simulink model "nonlinearGFLcontrol_shell"  (R2023b)
settings: Solver=VariableStepAuto  StartTime=0.0  StopTime=10.0  RelTol=1e-3
undefined symbols (not defined in the file or in its folder): freq, Ki_CC, ki_PLL, Kp_CC, kp_PLL, Lconv1
settings Model: Creator=weq968  LastModifiedBy=kauchr
settings DataIOCC: LoadExternalInput=on
settings RTWCC: GPUComputeCapability=5.0

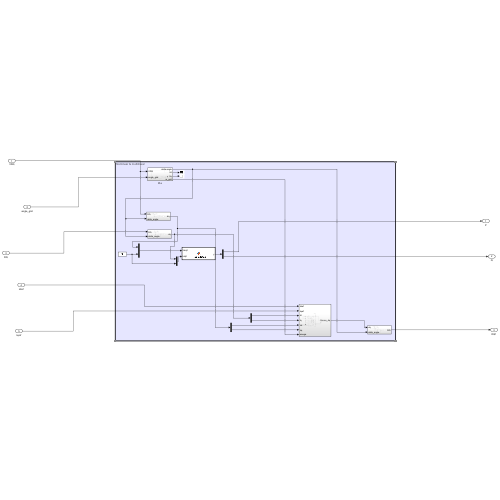
[thumbnail: Simulink's stored preview of the top-level diagram]
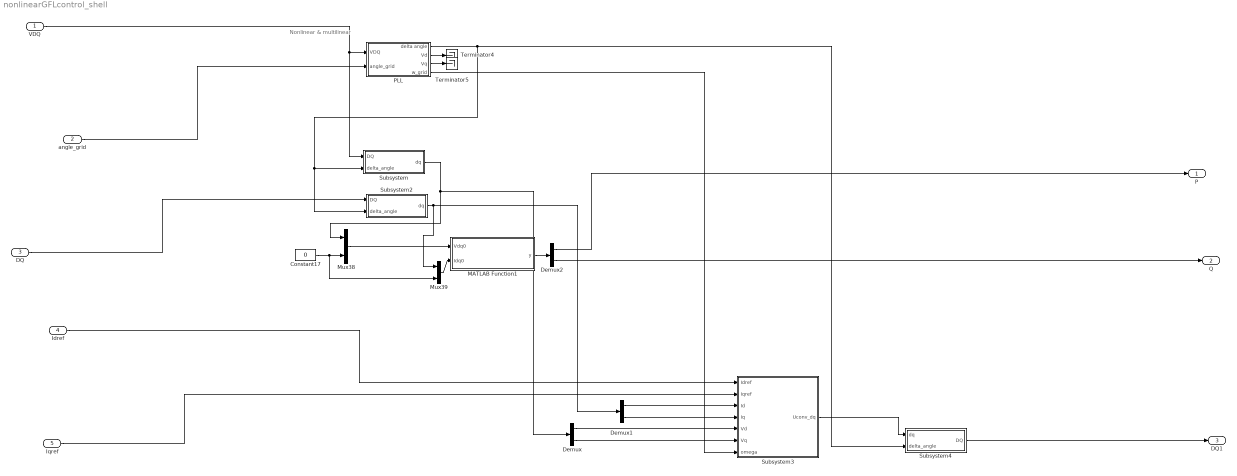
== system nonlinearGFLcontrol_shell ==
  note: Nonlinear & multilinear
  VDQ : Inport
  angle_grid : Inport  Port=2
  DQ : Inport  Port=3
  Idref : Inport  Port=4
  Iqref : Inport  Port=5
  Constant17 : Constant  Value=0
  Demux : Demux  Outputs=2
  Demux1 : Demux  Outputs=2
  Demux2 : Demux  Outputs=2
  MATLAB Function1 : MATLAB Function  TreatAsAtomicUnit=on
  Mux38 : Mux  Inputs=[2 1]
  Mux39 : Mux  Inputs=[2 1]
  PLL : Subsystem
  Subsystem : Subsystem
  Subsystem2 : Subsystem
  Subsystem3 : Subsystem
  Subsystem4 : Subsystem
  Terminator4 : Terminator
  Terminator5 : Terminator
  P : Outport
  Q : Outport  Port=2
  DQ1 : Outport  Port=3
  wires:
  Demux/1 -> Subsystem3/5(Vd)
  Demux1/1 -> Subsystem3/3(Id)
  PLL/4(w_grid) -> Subsystem3/7(omega)
  Subsystem3/1(Uconv_dq) -> Subsystem4/1(dq)
  PLL/2(Vd) -> Terminator4/1
  Iqref/1 -> Subsystem3/2(Iqref)
  Demux2/2 -> Q/1
  Subsystem4/1(DQ) -> DQ1/1
  Idref/1 -> Subsystem3/1(Idref)
  DQ/1 -> Subsystem2/1(DQ)
  Demux1/2 -> Subsystem3/4(Iq)
  Subsystem/1(dq) -> Mux38/1, Demux/1
  Subsystem2/1(dq) -> Mux39/1, Demux1/1
  angle_grid/1 -> PLL/2(angle_grid)
  PLL/1(delta angle) -> Subsystem2/2(delta_angle), Subsystem/2(delta_angle), Subsystem4/2(delta_angle)
  Constant17/1 -> Mux39/2, Mux38/2
  Demux/2 -> Subsystem3/6(Vq)
  VDQ/1 -> Subsystem/1(DQ), PLL/1(VDQ)
  Demux2/1 -> P/1
  Mux39/1 -> MATLAB Function1/2(Idq0)
  Mux38/1 -> MATLAB Function1/1(Vdq0)
  PLL/3(Vq) -> Terminator5/1
  MATLAB Function1/1(y) -> Demux2/1

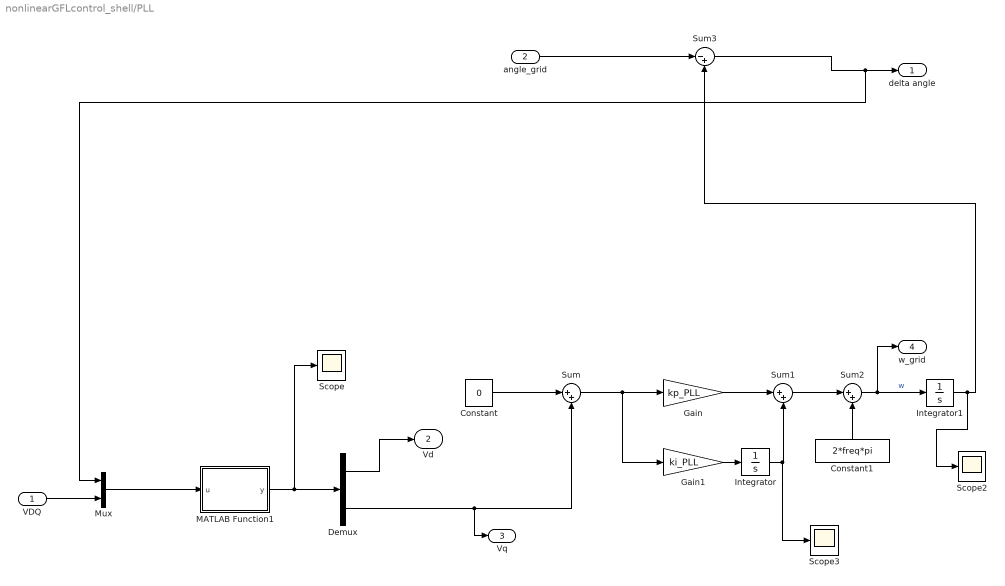
== system nonlinearGFLcontrol_shell/PLL ==
  VDQ : Inport
  angle_grid : Inport  Port=2
  Constant : Constant  Value=0
  Constant1 : Constant  Value=2*freq*pi
  Demux : Demux  Outputs=2
  Gain : Gain  Gain=kp_PLL
  Gain1 : Gain  Gain=ki_PLL
  Integrator : Integrator  ContinuousStateAttributes='converter2_xI_PLL'
  Integrator1 : Integrator  ContinuousStateAttributes='converter2_thetaPLL'
  MATLAB Function1 : MATLAB Function  TreatAsAtomicUnit=on
  Mux : Mux  Inputs=[1 2]
  Scope : Scope
  Scope2 : Scope
  Scope3 : Scope
  Sum : Sum  Inputs=|++
  Sum1 : Sum  Inputs=|++
  Sum2 : Sum  Inputs=|++
  Sum3 : Sum  Inputs=|-+
  delta angle : Outport
  Vd : Outport  Port=2
  Vq : Outport  Port=3
  w_grid : Outport  Port=4
  wires:
  Sum1/1 -> Sum2/1
  Gain/1 -> Sum1/1
  Integrator/1 -> Scope3/1, Sum1/2
  Gain1/1 -> Integrator/1
  Demux/1 -> Vd/1
  Sum2/1 -> w_grid/1, Integrator1/1  "w"
  Constant/1 -> Sum/1
  Constant1/1 -> Sum2/2
  MATLAB Function1/1(y) -> Scope/1, Demux/1
  VDQ/1 -> Mux/2
  Sum/1 -> Gain1/1, Gain/1
  Mux/1 -> MATLAB Function1/1(u)
  Demux/2 -> Vq/1, Sum/2
  Integrator1/1 -> Scope2/1, Sum3/2
  Sum3/1 -> Mux/1, delta angle/1
  angle_grid/1 -> Sum3/1

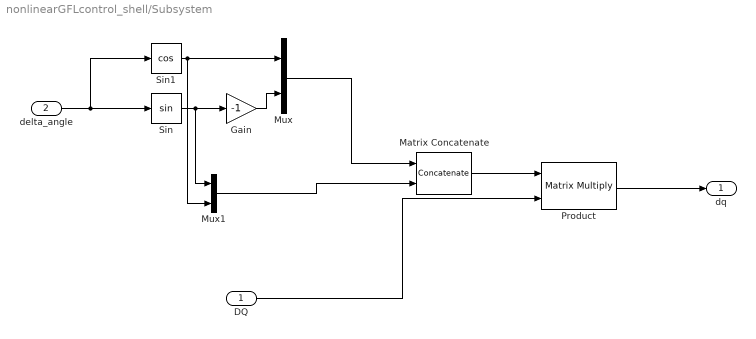
== system nonlinearGFLcontrol_shell/Subsystem ==
  DQ : Inport
  delta_angle : Inport  Port=2
  Gain : Gain  Gain=-1
  Matrix Concatenate : Concatenate  Mode=Multidimensional array  ConcatenateDimension=2
  Mux : Mux  Inputs=2
  Mux1 : Mux  Inputs=2
  Product : Product  Multiplication=Matrix(*)
  Sin : Trigonometry
  Sin1 : Trigonometry  Operator=cos
  dq : Outport
  wires:
  Matrix Concatenate/1 -> Product/1
  DQ/1 -> Product/2
  Product/1 -> dq/1
  delta_angle/1 -> Sin1/1, Sin/1
  Sin1/1 -> Mux1/2, Mux/1
  Sin/1 -> Mux1/1, Gain/1
  Gain/1 -> Mux/2
  Mux/1 -> Matrix Concatenate/1
  Mux1/1 -> Matrix Concatenate/2

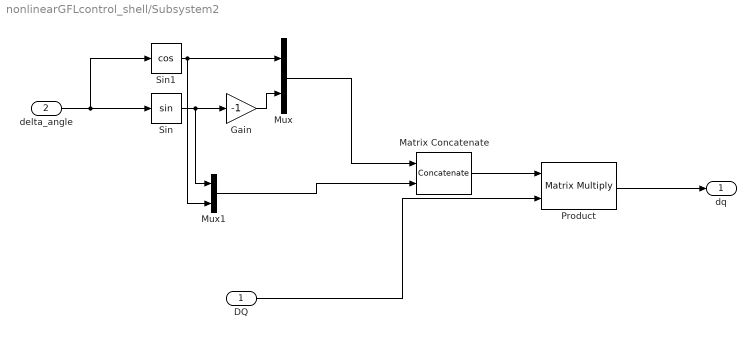
== system nonlinearGFLcontrol_shell/Subsystem2 ==
  DQ : Inport
  delta_angle : Inport  Port=2
  Gain : Gain  Gain=-1
  Matrix Concatenate : Concatenate  Mode=Multidimensional array  ConcatenateDimension=2
  Mux : Mux  Inputs=2
  Mux1 : Mux  Inputs=2
  Product : Product  Multiplication=Matrix(*)
  Sin : Trigonometry
  Sin1 : Trigonometry  Operator=cos
  dq : Outport
  wires:
  Matrix Concatenate/1 -> Product/1
  DQ/1 -> Product/2
  Product/1 -> dq/1
  delta_angle/1 -> Sin1/1, Sin/1
  Sin1/1 -> Mux1/2, Mux/1
  Sin/1 -> Mux1/1, Gain/1
  Gain/1 -> Mux/2
  Mux/1 -> Matrix Concatenate/1
  Mux1/1 -> Matrix Concatenate/2

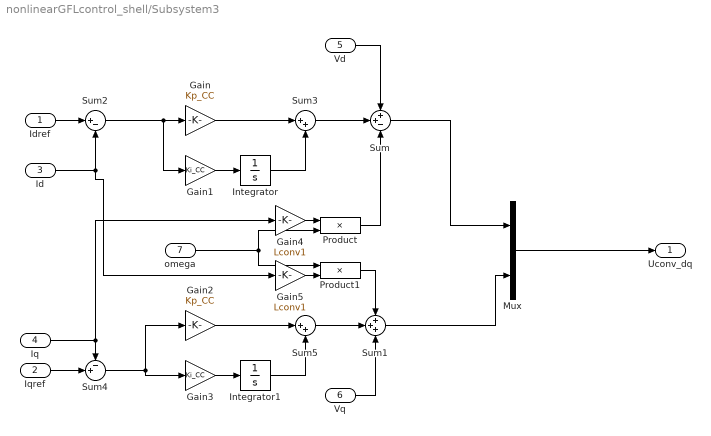
== system nonlinearGFLcontrol_shell/Subsystem3 ==
  Idref : Inport
  Iqref : Inport  Port=2
  Id : Inport  Port=3
  Iq : Inport  Port=4
  Vd : Inport  Port=5
  Vq : Inport  Port=6
  omega : Inport  Port=7
  Gain : Gain  Gain=Kp_CC
  Gain1 : Gain  Gain=Ki_CC
  Gain2 : Gain  Gain=Kp_CC
  Gain3 : Gain  Gain=Ki_CC
  Gain4 : Gain  Gain=Lconv1
  Gain5 : Gain  Gain=Lconv1
  Integrator : Integrator  ContinuousStateAttributes='converter2_xId_CC'
  Integrator1 : Integrator  ContinuousStateAttributes='converter2_xIq_CC'
  Mux : Mux  Inputs=2
  Product : Product
  Product1 : Product
  Sum : Sum  Inputs=++-
  Sum1 : Sum  Inputs=+++
  Sum2 : Sum  Inputs=|+-
  Sum3 : Sum  Inputs=|++
  Sum4 : Sum  Inputs=-+|
  Sum5 : Sum  Inputs=|++
  Uconv_dq : Outport
  wires:
  Vd/1 -> Sum/1
  Vq/1 -> Sum1/3
  Sum/1 -> Mux/1
  Sum1/1 -> Mux/2
  Mux/1 -> Uconv_dq/1
  Idref/1 -> Sum2/1
  Id/1 -> Sum2/2, Gain5/1
  Sum2/1 -> Gain1/1, Gain/1
  Gain1/1 -> Integrator/1
  Integrator/1 -> Sum3/2
  Gain/1 -> Sum3/1
  Sum3/1 -> Sum/2
  Iqref/1 -> Sum4/2
  Iq/1 -> Gain4/1, Sum4/1
  Integrator1/1 -> Sum5/2
  Sum5/1 -> Sum1/2
  Gain3/1 -> Integrator1/1
  Gain2/1 -> Sum5/1
  Sum4/1 -> Gain2/1, Gain3/1
  Gain4/1 -> Product/1
  Product/1 -> Sum/3
  omega/1 -> Product/2, Product1/1
  Gain5/1 -> Product1/2
  Product1/1 -> Sum1/1

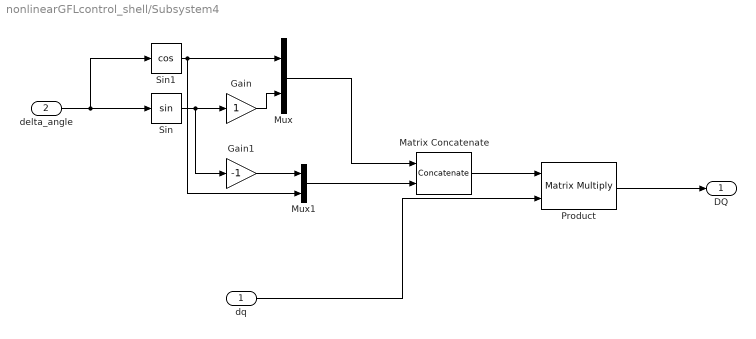
== system nonlinearGFLcontrol_shell/Subsystem4 ==
  dq : Inport
  delta_angle : Inport  Port=2
  Gain : Gain
  Gain1 : Gain  Gain=-1
  Matrix Concatenate : Concatenate  Mode=Multidimensional array  ConcatenateDimension=2
  Mux : Mux  Inputs=2
  Mux1 : Mux  Inputs=2
  Product : Product  Multiplication=Matrix(*)
  Sin : Trigonometry
  Sin1 : Trigonometry  Operator=cos
  DQ : Outport
  wires:
  Matrix Concatenate/1 -> Product/1
  dq/1 -> Product/2
  Product/1 -> DQ/1
  delta_angle/1 -> Sin1/1, Sin/1
  Sin1/1 -> Mux1/2, Mux/1
  Sin/1 -> Gain1/1, Gain/1
  Gain/1 -> Mux/2
  Mux/1 -> Matrix Concatenate/1
  Mux1/1 -> Matrix Concatenate/2
  Gain1/1 -> Mux1/1

== matlab function nonlinearGFLcontrol_shell/PLL/MATLAB Function1 ==
  data: u input; y output
function y = DQ2dq(u)
 
y =([cos(u(1)), sin(u(1)); -sin(u(1)), cos(u(1))])*[u(2);u(3)];

== matlab function nonlinearGFLcontrol_shell/MATLAB Function1 ==
  data: Vdq0 input; y output; Idq0 input
function y = PQcalculation(Vdq0,Idq0)
 % alignment with d-axis
y =3/2*([Vdq0(1)*Idq0(1)+Vdq0(2)*Idq0(2)+2*Vdq0(3)*Idq0(3);Vdq0(2)*Idq0(1)-Vdq0(1)*Idq0(2);]);
